simulink model "MIL_ASW"  (R2019b)
settings: Solver=FixedStepDiscrete  StartTime=0.0  StopTime=2  FixedStep=0.001  RelTol=1e-3  EnableMultiTasking=on
model workspace (MAT data in the model file):
  AccPedlCanVal : Simulink.Signal (value not decoded)
  AccPedlVal : Simulink.Signal (value not decoded)
  BrkPedlCanVal : Simulink.Signal (value not decoded)
  BrkPedlVal : Simulink.Signal (value not decoded)
  Cal1 : Simulink.Parameter (value not decoded)
  Cal10 : Simulink.Parameter (value not decoded)
  Cal11 : Simulink.Parameter (value not decoded)
  Cal12 : Simulink.Parameter (value not decoded)
  Cal2 : Simulink.Parameter (value not decoded)
  Cal3 : Simulink.Parameter (value not decoded)
  Cal4 : Simulink.Parameter (value not decoded)
  Cal5 : Simulink.Parameter (value not decoded)
  Cal6 : Simulink.Parameter (value not decoded)
  Cal7 : Simulink.Parameter (value not decoded)
  Cal8 : Simulink.Parameter (value not decoded)
  Cal9 : Simulink.Parameter (value not decoded)
  Clu1Act : Simulink.Signal (value not decoded)
  Clu1PTar : Simulink.Signal (value not decoded)
  Clu1Req : Simulink.Signal (value not decoded)
  Clu1TqTar : Simulink.Signal (value not decoded)
  Clu2Act : Simulink.Signal (value not decoded)
  Clu2PTar : Simulink.Signal (value not decoded)
  Clu2Req : Simulink.Signal (value not decoded)
  Clu2TqTar : Simulink.Signal (value not decoded)
  CluKissPtPLnch : Simulink.Parameter (value not decoded)
  CluOilTRawVal : Simulink.Signal (value not decoded)
  CluOilTVal : Simulink.Signal (value not decoded)
  CluOpenTqRatMax : Simulink.Parameter (value not decoded)
  CluPMap : Simulink.Parameter (value not decoded)
  CluPMax : Simulink.Parameter (value not decoded)
  CluPMaxGear1 : Simulink.Parameter (value not decoded)
  CluPMaxGear2 : Simulink.Parameter (value not decoded)
  CluPMaxGear3 : Simulink.Parameter (value not decoded)
  CluPMaxGear4 : Simulink.Parameter (value not decoded)
  CluPMaxGear5 : Simulink.Parameter (value not decoded)
  CluPMaxGear6 : Simulink.Parameter (value not decoded)
  CluPMaxGearR : Simulink.Parameter (value not decoded)
  CluPMin : Simulink.Parameter (value not decoded)
  CluPosnMax : Simulink.Parameter (value not decoded)
  CluSoln1IRawVal : Simulink.Signal (value not decoded)
  CluSoln1IReq : Simulink.Signal (value not decoded)
  CluSoln1IReqFlg : Simulink.Signal (value not decoded)
  CluSoln1IVal : Simulink.Signal (value not decoded)
  CluSoln1LineI : Simulink.Parameter (value not decoded)
  CluSoln1LineP : Simulink.Parameter (value not decoded)
  CluSoln1Pwm : Simulink.Signal (value not decoded)
  CluSoln2IRawVal : Simulink.Signal (value not decoded)
  CluSoln2IReq : Simulink.Signal (value not decoded)
  CluSoln2IReqFlg : Simulink.Signal (value not decoded)
  CluSoln2IVal : Simulink.Signal (value not decoded)
  CluSoln2LineI : Simulink.Parameter (value not decoded)
  CluSoln2LineP : Simulink.Parameter (value not decoded)
  CluSoln2Pwm : Simulink.Signal (value not decoded)
  CluTqMap : Simulink.Parameter (value not decoded)
  CrnkSpdRawVal : Simulink.Signal (value not decoded)
  CrnkSpdVal : Simulink.Signal (value not decoded)
  Drive_Intensity_Fuzzy : object (value not decoded)
  DrvIntenFzzy : Simulink.LookupTable (value not decoded)
  EngNIdle : Simulink.Parameter (value not decoded)
  EngNIdleMin : Simulink.Parameter (value not decoded)
  EngSpdCanVal : Simulink.Signal (value not decoded)
  EngThrCanVal : Simulink.Signal (value not decoded)
  EngTqAdd : Simulink.Parameter (value not decoded)
  EngTqCanVal : Simulink.Signal (value not decoded)
  EngTqIntvFlg : Simulink.Signal (value not decoded)
  EngTqIntvRat : Simulink.Signal (value not decoded)
  EngTqMapExtChartc : Simulink.Parameter (value not decoded)
  EngTqMapSpdIndx : Simulink.Parameter (value not decoded)
  EngTqMapThrtIndx : Simulink.Parameter (value not decoded)
  EngTqMapTqMax : Simulink.Parameter (value not decoded)
  EngTqMaxNorm : Simulink.Parameter (value not decoded)
  EngTqRef : Simulink.Parameter (value not decoded)
  EvenCluPRawVal : Simulink.Signal (value not decoded)
  EvenCluPVal : Simulink.Signal (value not decoded)
  EvenInpSpdRawVal : Simulink.Signal (value not decoded)
  EvenInpSpdVal : Simulink.Signal (value not decoded)
  FcnCallTime : Simulink.Parameter (value not decoded)
  FinalRat : Simulink.Parameter (value not decoded)
  Fork1A : Simulink.Parameter (value not decoded)
  Fork1Act : Simulink.Signal (value not decoded)
  Fork1B : Simulink.Parameter (value not decoded)
  Fork1DeltaSpdTar : Simulink.Parameter (value not decoded)
  Fork1MaxSpd1A : Simulink.Parameter (value not decoded)
  Fork1MaxSpd1B : Simulink.Parameter (value not decoded)
  Fork1MaxSpd2A : Simulink.Parameter (value not decoded)
  Fork1MaxSpd2B : Simulink.Parameter (value not decoded)
  Fork1PosnA : Simulink.Parameter (value not decoded)
  Fork1PosnB : Simulink.Parameter (value not decoded)
  Fork1PosnMaxSpd1A : Simulink.Parameter (value not decoded)
  Fork1PosnMaxSpd1B : Simulink.Parameter (value not decoded)
  Fork1PosnMaxSpd2A : Simulink.Parameter (value not decoded)
  Fork1PosnMaxSpd2B : Simulink.Parameter (value not decoded)
  Fork1PosnNeut : Simulink.Parameter (value not decoded)
  Fork1PosnNeutA : Simulink.Parameter (value not decoded)
  Fork1PosnNeutB : Simulink.Parameter (value not decoded)
  Fork1PosnRawVal : Simulink.Signal (value not decoded)
  Fork1PosnSyncA : Simulink.Parameter (value not decoded)
  Fork1PosnSyncB : Simulink.Parameter (value not decoded)
  Fork1PosnVal : Simulink.Signal (value not decoded)
  Fork1SyncTar : Simulink.Parameter (value not decoded)
  Fork2A : Simulink.Parameter (value not decoded)
  Fork2Act : Simulink.Signal (value not decoded)
  Fork2B : Simulink.Parameter (value not decoded)
  Fork2DeltaSpdTar : Simulink.Parameter (value not decoded)
  Fork2MaxSpd1A : Simulink.Parameter (value not decoded)
  Fork2MaxSpd1B : Simulink.Parameter (value not decoded)
  Fork2MaxSpd2A : Simulink.Parameter (value not decoded)
  Fork2MaxSpd2B : Simulink.Parameter (value not decoded)
  Fork2PosnA : Simulink.Parameter (value not decoded)
  Fork2PosnB : Simulink.Parameter (value not decoded)
  Fork2PosnMaxSpd1A : Simulink.Parameter (value not decoded)
  Fork2PosnMaxSpd1B : Simulink.Parameter (value not decoded)
  Fork2PosnMaxSpd2A : Simulink.Parameter (value not decoded)
  Fork2PosnMaxSpd2B : Simulink.Parameter (value not decoded)
  Fork2PosnNeut : Simulink.Parameter (value not decoded)
  Fork2PosnNeutA : Simulink.Parameter (value not decoded)
  Fork2PosnNeutB : Simulink.Parameter (value not decoded)
  Fork2PosnRawVal : Simulink.Signal (value not decoded)
  Fork2PosnSyncA : Simulink.Parameter (value not decoded)
  Fork2PosnSyncB : Simulink.Parameter (value not decoded)
  Fork2PosnVal : Simulink.Signal (value not decoded)
  Fork2SyncTar : Simulink.Parameter (value not decoded)
  Fork3A : Simulink.Parameter (value not decoded)
  Fork3Act : Simulink.Signal (value not decoded)
  Fork3B : Simulink.Parameter (value not decoded)
  Fork3DeltaSpdTar : Simulink.Parameter (value not decoded)
  Fork3MaxSpd1A : Simulink.Parameter (value not decoded)
  Fork3MaxSpd1B : Simulink.Parameter (value not decoded)
  Fork3MaxSpd2A : Simulink.Parameter (value not decoded)
  Fork3MaxSpd2B : Simulink.Parameter (value not decoded)
  Fork3PosnA : Simulink.Parameter (value not decoded)
  Fork3PosnB : Simulink.Parameter (value not decoded)
  Fork3PosnMaxSpd1A : Simulink.Parameter (value not decoded)
  Fork3PosnMaxSpd1B : Simulink.Parameter (value not decoded)
  Fork3PosnMaxSpd2A : Simulink.Parameter (value not decoded)
  Fork3PosnMaxSpd2B : Simulink.Parameter (value not decoded)
  Fork3PosnNeut : Simulink.Parameter (value not decoded)
  Fork3PosnNeutA : Simulink.Parameter (value not decoded)
  Fork3PosnNeutB : Simulink.Parameter (value not decoded)
  Fork3PosnRawVal : Simulink.Signal (value not decoded)
  Fork3PosnSyncA : Simulink.Parameter (value not decoded)
  Fork3PosnSyncB : Simulink.Parameter (value not decoded)
  Fork3PosnVal : Simulink.Signal (value not decoded)
  Fork3SyncTar : Simulink.Parameter (value not decoded)
  Fork4A : Simulink.Parameter (value not decoded)
  Fork4Act : Simulink.Signal (value not decoded)
  Fork4B : Simulink.Parameter (value not decoded)
  Fork4DeltaSpdTar : Simulink.Parameter (value not decoded)
  Fork4MaxSpd1A : Simulink.Parameter (value not decoded)
  Fork4MaxSpd1B : Simulink.Parameter (value not decoded)
  Fork4MaxSpd2A : Simulink.Parameter (value not decoded)
  Fork4MaxSpd2B : Simulink.Parameter (value not decoded)
  Fork4PosnA : Simulink.Parameter (value not decoded)
  Fork4PosnB : Simulink.Parameter (value not decoded)
  Fork4PosnMaxSpd1A : Simulink.Parameter (value not decoded)
  Fork4PosnMaxSpd1B : Simulink.Parameter (value not decoded)
  Fork4PosnMaxSpd2A : Simulink.Parameter (value not decoded)
  Fork4PosnMaxSpd2B : Simulink.Parameter (value not decoded)
  Fork4PosnNeut : Simulink.Parameter (value not decoded)
  Fork4PosnNeutA : Simulink.Parameter (value not decoded)
  Fork4PosnNeutB : Simulink.Parameter (value not decoded)
  Fork4PosnRawVal : Simulink.Signal (value not decoded)
  Fork4PosnSyncA : Simulink.Parameter (value not decoded)
  Fork4PosnSyncB : Simulink.Parameter (value not decoded)
  Fork4PosnVal : Simulink.Signal (value not decoded)
  Fork4SyncTar : Simulink.Parameter (value not decoded)
  FrntWhlRd : Simulink.Parameter (value not decoded)
  GearIdx : Simulink.Parameter (value not decoded)
  GearMax : Simulink.Parameter (value not decoded)
  GearRat : Simulink.Parameter (value not decoded)
  Launch_Engage_Fuzzy : object (value not decoded)
  LnchEngmtFzzy : Simulink.LookupTable (value not decoded)
  LubeSolnIRawVal : Simulink.Signal (value not decoded)
  LubeSolnIReq : Simulink.Signal (value not decoded)
  LubeSolnIVal : Simulink.Signal (value not decoded)
  LubeSolnLineI : Simulink.Parameter (value not decoded)
  LubeSolnLineP : Simulink.Parameter (value not decoded)
  LubeSolnPwm : Simulink.Signal (value not decoded)
  MaiLineSolnIRawVal : Simulink.Signal (value not decoded)
  MaiLineSolnIReq : Simulink.Signal (value not decoded)
  MaiLineSolnIVal : Simulink.Signal (value not decoded)
  MaiLineSolnLineI : Simulink.Parameter (value not decoded)
  MaiLineSolnLineP : Simulink.Parameter (value not decoded)
  MaiLineSolnPwm : Simulink.Signal (value not decoded)
  OddCluPRawVal : Simulink.Signal (value not decoded)
  OddCluPVal : Simulink.Signal (value not decoded)
  OddInpSpdRawVal : Simulink.Signal (value not decoded)
  OddInpSpdVal : Simulink.Signal (value not decoded)
  OutpSpdRawVal : Simulink.Signal (value not decoded)
  OutpSpdVal : Simulink.Signal (value not decoded)
  PsnsrLineP : Simulink.Parameter (value not decoded)
  PsnsrLineV : Simulink.Parameter (value not decoded)
  SftLvrCanVal : Simulink.Signal (value not decoded)
  SftLvrCfm : Simulink.Signal (value not decoded)
  SftLvrVal : Simulink.Signal (value not decoded)
  Shaft1GearAct : Simulink.Signal (value not decoded)
  Shaft1GearReq : Simulink.Signal (value not decoded)
  Shaft2GearAct : Simulink.Signal (value not decoded)
  Shaft2GearReq : Simulink.Signal (value not decoded)
  ShiftMux1SwtReq : Simulink.Signal (value not decoded)
  ShiftMux2SwtReq : Simulink.Signal (value not decoded)
  ShiftSdlEcoDwnSeln : Simulink.Parameter (value not decoded)
  ShiftSdlEcoDwnShift : Simulink.Parameter (value not decoded)
  ShiftSdlEcoUpSeln : Simulink.Parameter (value not decoded)
  ShiftSdlEcoUpShift : Simulink.Parameter (value not decoded)
  ShiftSdlPwrDwnSeln : Simulink.Parameter (value not decoded)
  ShiftSdlPwrDwnShift : Simulink.Parameter (value not decoded)
  ShiftSdlPwrUpSeln : Simulink.Parameter (value not decoded)
  ShiftSdlPwrUpShift : Simulink.Parameter (value not decoded)
  ShiftSdlSACDwnSeln : Simulink.Parameter (value not decoded)
  ShiftSdlSACDwnShift : Simulink.Parameter (value not decoded)
  ShiftSdlSACUpSeln : Simulink.Parameter (value not decoded)
  ShiftSdlSACUpShift : Simulink.Parameter (value not decoded)
  ShiftSdlThrPedlIdx : Simulink.Parameter (value not decoded)
  ShiftSoln1IRawVal : Simulink.Signal (value not decoded)
  ShiftSoln1IReq : Simulink.Signal (value not decoded)
  ShiftSoln1IVal : Simulink.Signal (value not decoded)
  ShiftSoln1LineI : Simulink.Parameter (value not decoded)
  ShiftSoln1LineP : Simulink.Parameter (value not decoded)
  ShiftSoln1Pwm : Simulink.Signal (value not decoded)
  ShiftSoln2IRawVal : Simulink.Signal (value not decoded)
  ShiftSoln2IReq : Simulink.Signal (value not decoded)
  ShiftSoln2IVal : Simulink.Signal (value not decoded)
  ShiftSoln2LineI : Simulink.Parameter (value not decoded)
  ShiftSoln2LineP : Simulink.Parameter (value not decoded)
  ShiftSoln2Pwm : Simulink.Signal (value not decoded)
  SolnOutpTRawVal : Simulink.Signal (value not decoded)
  SolnOutpTVal : Simulink.Signal (value not decoded)
  TSnsr1LineR : Simulink.Parameter (value not decoded)
  TSnsr2LineR : Simulink.Parameter (value not decoded)
  TrsmNrGearAct : Simulink.Signal (value not decoded)
  TrsmNrGearReq : Simulink.Signal (value not decoded)
  TrsmNrPreGearAct : Simulink.Signal (value not decoded)
  TrsmNrPreGearReq : Simulink.Signal (value not decoded)
  Tsnsr1LineT : Simulink.Parameter (value not decoded)
  Tsnsr2LineT : Simulink.Parameter (value not decoded)
  VehSpdCanVal : Simulink.Signal (value not decoded)
  VehSpdTrsmEstimd : Simulink.Signal (value not decoded)
  VehSpdVal : Simulink.Signal (value not decoded)
  VlvBodyTRawVal : Simulink.Signal (value not decoded)
  VlvBodyTVal : Simulink.Signal (value not decoded)
symbols that are objects in the model workspace (value not decoded): CluPMap, CluSoln1LineI, CluSoln1LineP, CluSoln2LineI, CluSoln2LineP, CluTqMap, EngNIdle, EngNIdleMin, EngTqMapThrtIndx, EngTqMapTqMax, EngTqMaxNorm, FcnCallTime, FinalRat, Fork1A, Fork1B, Fork1DeltaSpdTar, Fork1PosnA, Fork1PosnB, Fork1PosnMaxSpd1A, Fork1PosnMaxSpd1B, Fork1PosnMaxSpd2A, Fork1PosnMaxSpd2B, Fork1PosnNeut, Fork1PosnNeutA, Fork1PosnNeutB, Fork1PosnSyncA, Fork1PosnSyncB, Fork1SyncTar, Fork2A, Fork2B, Fork2DeltaSpdTar, Fork2PosnA, Fork2PosnB, Fork2PosnMaxSpd1A, Fork2PosnMaxSpd1B, Fork2PosnMaxSpd2A, Fork2PosnMaxSpd2B, Fork2PosnNeut, Fork2PosnNeutA, Fork2PosnNeutB, Fork2PosnSyncA, Fork2PosnSyncB, Fork2SyncTar, Fork3A, Fork3B, Fork3DeltaSpdTar, Fork3PosnA, Fork3PosnB, Fork3PosnMaxSpd1A, Fork3PosnMaxSpd1B, Fork3PosnMaxSpd2A, Fork3PosnMaxSpd2B, Fork3PosnNeut, Fork3PosnNeutA, Fork3PosnNeutB, Fork3PosnSyncA, Fork3PosnSyncB, Fork3SyncTar, Fork4A, Fork4B
undefined symbols (not defined in the file or in its folder): in1, out1
libraries: simulink x44, fuzblock x3
(part 8 of 10)

== stateflow chart MIL_ASW/Application_Software_SHAW/TR_Scheduler/Scheduler ==
  (default) -> (junction 2)
  (junction 2) -> (junction 3) [order 1] : [FirstSample == 1]
  (junction 2) -> (junction 4) [order 2]
  (junction 3) -> (junction 5) : {
      | FirstSample = 0;
      | Fncall_If;
      | Fncall_DrvgStgy;
      | Fncall_ShaftAcsCtrl;
      | Fncall_ShaftCtrl;
      | Fncall_GearPosnr;
      | Fncall_GearPCtrl;
      | Fncall_CluCtrl;
      | Fncall_CluPCtrl;
      | Fncall_TqCtrl;
      | Fncall_MaiLineCtrl;
      | }
  (junction 11) -> (junction 12) [order 1] : [Task20ms_Counter == 20]
  (junction 5) -> (junction 11)
  (junction 4) -> (junction 5)
  (junction 11) -> (junction 13) [order 2] : {
      | Task20ms_Counter++;
      | }
  (junction 12) -> (junction 14) : {
      | Task20ms_Counter = 1;
      | }
  (junction 13) -> (junction 14)
  (junction 14) -> (junction 21)
  (junction 21) -> (junction 22) [order 1] : [Task100ms_Counter == 100]
  (junction 21) -> (junction 23) [order 2] : {
      | Task100ms_Counter++;
      | }
  (junction 22) -> (junction 24) : {
      | Task100ms_Counter = 1;
      | }
  (junction 23) -> (junction 24)
  (junction 24) -> (junction 30)
  (junction 30) -> (junction 31) [order 1] : [Task10ms_Counter == 10]
  (junction 30) -> (junction 32) [order 2] : {
      | Task10ms_Counter++;
      | }
  (junction 31) -> (junction 33) : {
      | Fncall_If;
      | Fncall_DrvgStgy;
      | Fncall_ShaftAcsCtrl;
      | Fncall_ShaftCtrl;
      | Fncall_GearPosnr;
      | Fncall_GearPCtrl;
      | Fncall_CluCtrl;
      | Fncall_CluPCtrl;
      | Fncall_TqCtrl;
      | Fncall_MaiLineCtrl;
      | Task10ms_Counter = 1;
      | }
  (junction 32) -> (junction 33)
  (junction 33) -> (junction 39)
  data: FirstSample local uint8 =1; Task20ms_Counter local uint8; Task100ms_Counter local uint8; Task10ms_Counter local uint8; Fixed_Point local fixdt(0,32,6); Fixed_Point1 local fixdt(0,32,4); Fixed_Point2 local fixdt(0,32,6)
  events: Fncall_If output FUNCTION_CALL_EVENT; Fncall_DrvgStgy output FUNCTION_CALL_EVENT; Fncall_ShaftAcsCtrl output FUNCTION_CALL_EVENT; Fncall_ShaftCtrl output FUNCTION_CALL_EVENT; Fncall_GearPosnr output FUNCTION_CALL_EVENT; Fncall_GearPCtrl output FUNCTION_CALL_EVENT; Fncall_CluCtrl output FUNCTION_CALL_EVENT; Fncall_CluPCtrl output FUNCTION_CALL_EVENT; Fncall_TqCtrl output FUNCTION_CALL_EVENT; Fncall_MaiLineCtrl output FUNCTION_CALL_EVENT

== stateflow chart MIL_ASW/Application_Software_SHAW/ASW_DrivingStrategy/Auto_Mode_Decision/TrsmNrGearTarCalcnAutMod ==
  state Stop
    en:TrsmNrGearTarAutMod=0;
  state GearTarCalcn [function]
    (default) -> (junction 85)
    (junction 85) -> (junction 86) [order 1] : [TrsmNrGearAct==0&&...
        | ShiftLvrVal==3&&...
        | TrsmNrPreGearAct==1]
    (junction 86) -> (junction 97) : {TrsmNrGearTarAutMod=1;}
    (junction 85) -> (junction 87) [order 2]
    (junction 97) -> (junction 96)
    (junction 87) -> (junction 88) [order 1] : [TrsmNrGearAct==0&&...
        | ShiftLvrVal==1&&...
        | TrsmNrPreGearAct==7]
    (junction 88) -> (junction 96) : {TrsmNrGearTarAutMod=7;}
    (junction 87) -> (junction 89) [order 2]
    (junction 96) -> (junction 95)
    (junction 89) -> (junction 117) [order 1] : [(TrsmNrGearAct>0&&TrsmNrGearAct<7)&&...
        | ShiftLvrVal==3&&...
        | VehSpd<VehSpdDwnShift]
    (junction 117) -> (junction 90) [order 1] : [TrsmNrGearAct==TrsmNrPreGearAct+1]
    (junction 90) -> (junction 95) : {TrsmNrGearTarAutMod=TrsmNrGearAct-1;}
    (junction 89) -> (junction 92) [order 2]
    (junction 117) -> (junction 125) [order 2]
    (junction 95) -> (junction 129)
    (junction 125) -> (junction 127) : [TrsmNrGearAct==TrsmNrPreGearAct+2]
    (junction 127) -> (junction 129) : {TrsmNrGearTarAutMod=TrsmNrGearAct-2;}
    (junction 129) -> (junction 93)
    (junction 132) -> (junction 93) : {TrsmNrGearTarAutMod=TrsmNrGearAct+1;}
    (junction 134) -> (junction 132) [order 1] : [TrsmNrGearAct+1==TrsmNrPreGearAct]
    (junction 92) -> (junction 147) [order 1] : [(TrsmNrGearAct>0&&TrsmNrGearAct<7)&&...
        | ShiftLvrVal==3&&...
        | VehSpd>VehSpdUpShift]
    (junction 147) -> (junction 134) [order 2]
    (junction 93) -> (junction 140)
    (junction 134) -> (junction 135) [order 2]
    (junction 92) -> (junction 94) [order 2]
    (junction 147) -> (junction 149) [order 1] : [Upshift_Frozen(AccPedl,BrkVal,VehSpd)==1]
    (junction 135) -> (junction 139) : [TrsmNrGearAct+2==TrsmNrPreGearAct]
    (junction 139) -> (junction 140) : {TrsmNrGearTarAutMod=TrsmNrGearAct+2;}
    (junction 140) -> (junction 150)
    (junction 149) -> (junction 150)
    (junction 150) -> (junction 122)
    (junction 94) -> (junction 122)
  state flag=Upshift_Frozen(acc_pedl,brk_pedl,veh_spd) [function]
  state Fwd
    en:TrsmNrGearTarAutMod=TrsmNrPreGearAct;
    en,du:GearTarCalcn();
  (default) -> Stop
  Stop -> Fwd : [(ShiftLvrVal==3||ShiftLvrVal==1)&&...
      | BrkSig==0&&...
      | EngN>=EngNIdle*7/10]
  Fwd -> Stop : [(ShiftLvrVal!=3&&ShiftLvrVal!=1)||...
      | BrkSig==1||...
      | EngN<EngNIdle*7/10]
  data: acc_pedl function_input uint8; brk_pedl function_input uint8; veh_spd function_input uint16; flag function_output uint8; AccPedl input; ShiftLvrVal input; BrkVal input; BrkSig input; EngN input; TrsmNrGearAct input; TrsmNrPreGearAct input; VehSpd input; VehSpdUpShift input; VehSpdDwnShift input; TrsmNrGearTarAutMod output uint8; EngNIdle parameter uint16

== stateflow chart MIL_ASW/Application_Software_SHAW/ASW_DrivingStrategy/Auto_Mode_Decision/TrsmNrPreGearTarCalcnAutMod ==
  state Stop
    en:TrsmNrPreGearTarAutMod=0;
  state PreGearTarCalcn [function]
    (default) -> (junction 99)
    (junction 99) -> (junction 100) [order 1] : [TrsmNrGearAct==0&&ShiftLvrVal==3]
    (junction 100) -> (junction 111) : {TrsmNrPreGearTarAutMod=1;}
    (junction 99) -> (junction 101) [order 2]
    (junction 111) -> (junction 109)
    (junction 180) -> (junction 167) : {CntrR--;}
    (junction 102) -> (junction 180) [order 2]
    (junction 167) -> (junction 169)
    (junction 101) -> (junction 102) [order 1] : [TrsmNrGearAct==0&&ShiftLvrVal==1]
    (junction 102) -> (junction 169) [order 1] : [CntrR<=0]
        | {TrsmNrPreGearTarAutMod=7;
        | CntrR=50;}
    (junction 169) -> (junction 110)
    (junction 101) -> (junction 103) [order 2]
    (junction 110) -> (junction 182)
    (junction 103) -> (junction 104) [order 1] : [ShiftLvrVal==3&&...
        | VehSpd<VehSpdDwnSeln]
    (junction 104) -> (junction 109) : {TrsmNrPreGearTarAutMod=TrsmNrPreGearAct-1;}
    (junction 103) -> (junction 106) [order 2]
    (junction 109) -> (junction 107)
    (junction 106) -> (junction 105) [order 1] : [ShiftLvrVal==3&&...
        | VehSpd>VehSpdUpSeln]
    (junction 105) -> (junction 107) : {TrsmNrPreGearTarAutMod=TrsmNrPreGearAct+1;}
    (junction 106) -> (junction 108) [order 2]
    (junction 107) -> (junction 162)
    (junction 108) -> (junction 162)
    (junction 162) -> (junction 182) : {CntrR=50;}
  state Fwd
    en:TrsmNrPreGearTarAutMod=TrsmNrPreGearAct;
    en,du:PreGearTarCalcn();
  (default) -> Stop
  Stop -> Fwd : [ShiftLvrVal==3||ShiftLvrVal==1]
  Fwd -> Stop : [~(ShiftLvrVal==3||ShiftLvrVal==1)]
  data: CntrR local uint8 =50; ShiftLvrVal input; BrkVal input; BrkSig input; EngN input; TrsmNrGearAct input; TrsmNrPreGearAct input; VehSpd input; VehSpdUpSeln input; VehSpdDwnSeln input; TrsmNrPreGearTarAutMod output uint8; EngNIdle parameter uint16

== stateflow chart MIL_ASW/Application_Software_SHAW/ASW_GearPositioner/Fork1 ==
  state PosnTar = PosnTar(PosnAct) [function]
  state ForkAct = Ini_ForkAct(PosnAct) [function]
  state Initialization
    en:
    Fork1DirReq=0;
    Fork1PosnReq=Fork1PosnVal;
    du:
    Fork1ActLoc=Ini_ForkAct(Fork1PosnVal);
    ex:
    Fork1PosnReq=Fork1PosnVal;
  state error1
  state error
  state PositionBEngage
    state Phase1
      en,du:
      Fork1SyncPha=1;
      Fork1PosnReq=Fork1PosnVal-PosnTar(Fork1PosnVal);
    state Phase2
      en,du:
      Fork1SyncPha=2;
      Fork1DeltaSpdAct=Fork1BDeltaSpdAct;
      Fork1DeltaSpdReq=Fork1DeltaSpdAct-Fork1DeltaSpdTar*FcnCallTime;
    state Phase3
      en,du:
      Fork1SyncPha=3;
      Fork1PosnReq=Fork1PosnVal-PosnTar(Fork1PosnVal);
    PositionBEngage.Phase1 -> PositionBEngage.Phase2 : [Fork1PosnReq<=Fork1PosnSyncB]
    PositionBEngage.Phase2 -> PositionBEngage.Phase3 : [Fork1DeltaSpdAct<=Fork1SyncTar]
  state PositionAEngage
    state Phase1
      en,du:
      Fork1SyncPha=1;
      Fork1PosnReq=Fork1PosnVal+PosnTar(Fork1PosnVal);
    state Phase2
      en,du:
      Fork1SyncPha=2;
      Fork1DeltaSpdAct=Fork1ADeltaSpdAct;
      Fork1DeltaSpdReq=Fork1DeltaSpdAct-Fork1DeltaSpdTar*FcnCallTime;
    state Phase3
      en,du:
      Fork1SyncPha=3;
      Fork1PosnReq=Fork1PosnVal+PosnTar(Fork1PosnVal);
    PositionAEngage.Phase1 -> PositionAEngage.Phase2 : [Fork1PosnVal>=Fork1PosnSyncA]
    PositionAEngage.Phase2 -> PositionAEngage.Phase3 : [Fork1DeltaSpdAct<=Fork1SyncTar]
  state PositionADisengage
    state Phase1
      en:
      Fork1SyncPha=4;
      Fork1PosnReq=Fork1PosnNeut;
  state PositionBDisengage
    state Phase1
      en:
      Fork1SyncPha=4;
      Fork1PosnReq=Fork1PosnNeut;
  state Finish
    en:
    Fork1DirReq=0;
    Fork1ActLoc=Fork1ReqLoc;
    Fork1Act=Fork1ReqLoc;
  state Finish1
    en:
    Fork1DirReq=0;
    Fork1ActLoc=Fork1ReqLoc;
    Fork1Act=Fork1ReqLoc;
  (default) -> Initialization
  (junction 105) -> Initialization
  (junction 145) -> Initialization
  (junction 183) -> (junction 105)
  (junction 177) -> (junction 145)
  Initialization -> (junction 19) : [Fork1Req!=Fork1ActLoc]{Fork1ReqLoc=Fork1Req;}
  error -> (junction 177)
  (junction 21) -> error1 [order 3] : [Fork1ActLoc!=0]
  (junction 19) -> (junction 21) [order 2]
  (junction 19) -> (junction 22) [order 1] : [Fork1ReqLoc==0]
  (junction 22) -> error [order 3]
  error1 -> (junction 183)
  (junction 146) -> (junction 177)
  (junction 22) -> (junction 132) [order 1] : [Fork1ActLoc==Fork1A||...
      | Fork1ActLoc==Fork1A*10]
  (junction 21) -> (junction 27) [order 2] : [Fork1ReqLoc==Fork1B]
  (junction 21) -> (junction 72) [order 1] : [Fork1ReqLoc==Fork1A]
  (junction 22) -> (junction 131) [order 2] : [Fork1ActLoc==Fork1B||...
      | Fork1ActLoc==Fork1B*10]
  (junction 106) -> (junction 183)
  (junction 27) -> PositionBEngage.Phase1 : {Fork1DirReq=3;}
  (junction 131) -> PositionBDisengage.Phase1 : {Fork1DirReq=2;}
  (junction 72) -> PositionAEngage.Phase1 : {Fork1DirReq=1;}
  (junction 132) -> PositionADisengage.Phase1 : {Fork1DirReq=4;}
  Finish -> (junction 106)
  Finish1 -> (junction 146)
  PositionBEngage.Phase3 -> Finish : [Fork1PosnVal<=Fork1PosnB]
      | {Fork1SyncPha=4;}
  PositionADisengage.Phase1 -> Finish1 : [Fork1PosnVal<=Fork1PosnNeutA]
      | {Fork1SyncPha=0;}
  PositionAEngage.Phase3 -> Finish : [Fork1PosnVal>=Fork1PosnA]
      | {Fork1SyncPha=4;}
  PositionBDisengage.Phase1 -> Finish1 : [Fork1PosnVal>=Fork1PosnNeutB]
      | {Fork1SyncPha=0;}
  data: PosnTar function_output; PosnAct function_input uint16; PosnAct function_input uint16; ForkAct function_output; Fork1DirReq output uint8; Fork1SyncPha output uint8; Fork1DeltaSpdReq output uint16; Fork1PosnReq output uint16; Fork1DeltaSpdAct output uint16; Fork1Req input uint8; Fork1Act output uint8; Fork1PosnVal input uint16; Fork1ADeltaSpdAct input uint16; Fork1A parameter uint8; Fork1B parameter uint8; Fork1PosnSyncA parameter uint16; Fork1PosnSyncB parameter uint16; Fork1SyncTar parameter uint16; Fork1ReqLoc local uint8; Fork1DeltaSpdTar parameter uint16; FcnCallTime parameter uint8; Fork1PosnA parameter uint16; Fork1PosnB parameter uint16; Fork1PosnNeut parameter uint16; Fork1PosnNeutB parameter uint16; Fork1PosnNeutA parameter uint16; Fork1BDeltaSpdAct input uint16; Fork1ActLoc local uint8

== stateflow chart MIL_ASW/Application_Software_SHAW/ASW_GearPressureControl/Shift Actuate Valve Logic ==
  state Initial
    en:
    ShiftSoln1PReq= uint16(0);
    ShiftSoln2PReq= uint16(0);
  state ToGear1_OffGear3
    en,du:
    ShiftSoln1PReq= Fork1P*uint16(1)+uint16(500);
    ShiftSoln2PReq=Fork1P*uint16(2)+uint16(500);
  state ToGear3_OffGear1
    en,du:
    ShiftSoln1PReq= Fork1P*uint16(2)+uint16(500);
    ShiftSoln2PReq= Fork1P*uint16(1)+uint16(500);
  state ToGear2_OffGear4
    en,du:
    ShiftSoln1PReq= Fork2P*uint16(2)+uint16(500);
    ShiftSoln2PReq= Fork2P*uint16(1)+uint16(500);
  state ToGear4_OffGear2
    en,du:
    ShiftSoln1PReq= Fork2P*uint16(1)+uint16(500);
    ShiftSoln2PReq= Fork2P*uint16(2)+uint16(500);
  state OffGear5
    en,du:
    ShiftSoln1PReq= Fork3P*uint16(1)+uint16(500);
    ShiftSoln2PReq= Fork3P*uint16(2)+uint16(500);
  state ToGear5
    en,du:
    ShiftSoln1PReq= Fork3P*uint16(2)+uint16(500);
    ShiftSoln2PReq= Fork3P*uint16(1)+uint16(500);
  state ToGear6_OffRvs
    en,du:
    ShiftSoln1PReq= Fork4P*uint16(1)+uint16(500);
    ShiftSoln2PReq= Fork4P*uint16(2)+uint16(500);
  state ToRvs_OffGear6
    en,du:
    ShiftSoln1PReq= Fork4P*uint16(2)+uint16(500);
    ShiftSoln2PReq= Fork4P*uint16(1)+uint16(500);
  (default) -> Initial
  (junction 49) -> Initial
  (junction 30) -> (junction 49)
  Initial -> (junction 11)
  (junction 11) -> (junction 80) [order 1] : [Fork1Dir~=0]
      | {ShiftMux1SwtReq= uint8(0);
      | ShiftMux2SwtReq= uint8(0);}
  (junction 80) -> ToGear1_OffGear3 [order 1] : [Fork1Dir==1||Fork1Dir==2]
  ToGear1_OffGear3 -> (junction 30) : [Fork1Dir==0]
  (junction 11) -> (junction 43) [order 2]
  (junction 80) -> (junction 81) [order 2]
  (junction 32) -> (junction 30)
  (junction 81) -> ToGear3_OffGear1 : %[Fork1Dir==3||Fork1Dir==4]
  ToGear3_OffGear1 -> (junction 32) : [Fork1Dir==0]
  (junction 40) -> (junction 32)
  (junction 43) -> (junction 84) [order 1] : [Fork2Dir~=0]
      | {ShiftMux1SwtReq= uint8(1);
      | ShiftMux2SwtReq= uint8(1);}
  (junction 84) -> ToGear2_OffGear4 [order 1] : [Fork2Dir==1||Fork2Dir==2]
  ToGear2_OffGear4 -> (junction 40) : [Fork2Dir==0]
  (junction 43) -> (junction 60) [order 2]
  (junction 84) -> (junction 85) [order 2]
  (junction 39) -> (junction 40)
  (junction 85) -> ToGear4_OffGear2 : %[Fork2Dir==3||Fork2Dir==4]
  ToGear4_OffGear2 -> (junction 39) : [Fork2Dir==0]
  (junction 62) -> (junction 39)
  (junction 60) -> (junction 88) [order 1] : [Fork3Dir~=0]
      | {ShiftMux1SwtReq= uint8(1);
      | ShiftMux2SwtReq= uint8(0);}
  (junction 88) -> OffGear5 [order 1] : [Fork3Dir==1||Fork3Dir==2]
  OffGear5 -> (junction 62) : [Fork3Dir==0]
  (junction 60) -> (junction 73) [order 2]
  (junction 88) -> (junction 89) [order 2]
  (junction 63) -> (junction 62)
  (junction 89) -> ToGear5 : %[Fork3Dir==3||Fork3Dir==4]
  ToGear5 -> (junction 63) : [Fork3Dir==0]
  (junction 75) -> (junction 63)
  (junction 73) -> (junction 91) : [Fork4Dir~=0]
      | {ShiftMux1SwtReq= uint8(0);
      | ShiftMux2SwtReq= uint8(1);}
  (junction 91) -> ToGear6_OffRvs [order 1] : [Fork4Dir==1||Fork4Dir==2]
  ToGear6_OffRvs -> (junction 75) : [Fork4Dir==0]
  (junction 91) -> (junction 92) [order 2]
  (junction 79) -> (junction 75)
  (junction 92) -> ToRvs_OffGear6 : %[Fork4Dir==3||Fork4Dir==4]
  ToRvs_OffGear6 -> (junction 79) : [Fork4Dir==0]
  data: Fork1Dir input uint8; Fork1P input uint16; Fork2Dir input uint8; Fork2P input uint16; Fork3Dir input uint8; Fork3P input uint16; Fork4Dir input uint8; ShiftMux1SwtReq output uint8; ShiftMux2SwtReq output uint8; ShiftSoln1PReq output uint16; ShiftSoln2PReq output uint16; Fork4P input uint16
